simulink model "s3_c2_luenberger"  (R2023a)
settings: Solver=FixedStepAuto  StartTime=0.0  StopTime=32  FixedStep=1E-3  RelTol=1e-3
undefined symbols (not defined in the file): A, A_c2, B1, C, C_obs1, C_obs2, CI, Ko1_luenberger, Ko2_luenberger
settings Model: Creator=felipe  LastModifiedBy=felipe

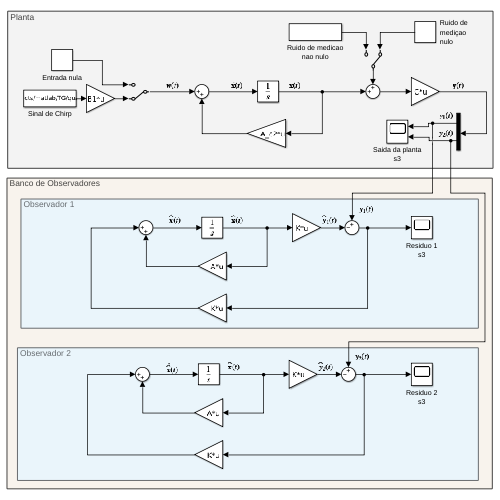
[thumbnail: Simulink's stored preview of the top-level diagram]
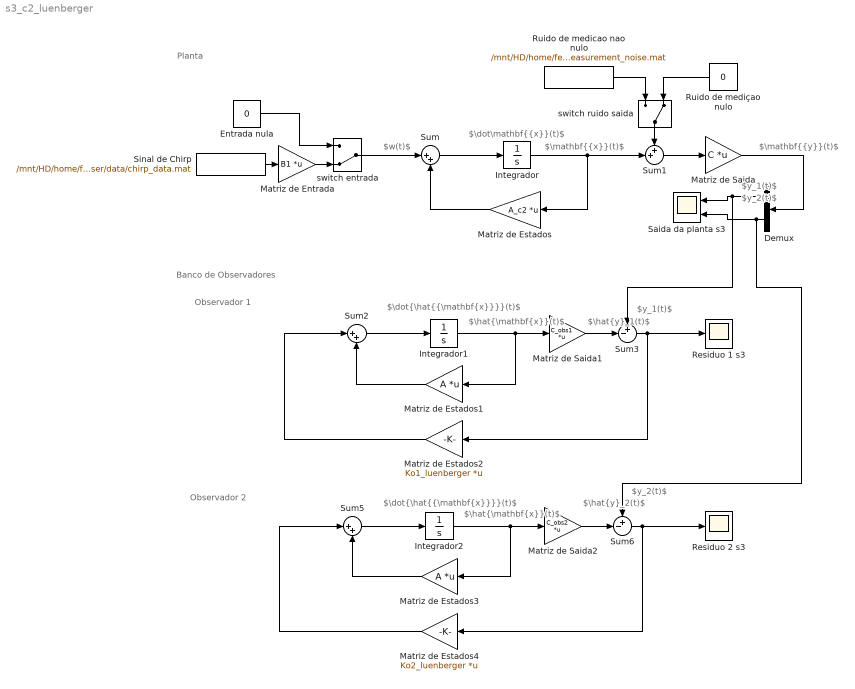
== system s3_c2_luenberger ==
  note: $\dot{\hat{{\mathbf{x}}}}(t)$
  note: Banco de Observadores
  note: Observador 1
  note: $w(t)$
  note: Planta
  note: $\dot\mathbf{{x}}(t)$
  note: $\mathbf{{x}}(t)$
  note: $\mathbf{{y}}(t)$
  note: Observador 2
  note: $y_1(t)$
  note: $y_2(t)$
  note: $\hat{y}_1(t)$
  note: $\hat{\mathbf{x}}(t)$
  note: $\dot{\hat{{\mathbf{x}}}}(t)$
  note: $\hat{y}_2(t)$
  note: $\hat{\mathbf{x}}(t)$
  note: $y_1(t)$
  note: $y_2(t)$
  Demux : Demux  Outputs=2
  Entrada nula : Constant  Value=0
  Integrador : Integrator  InitialCondition=CI
  Integrador1 : Integrator
  Integrador2 : Integrator
  Matriz de Entrada : Gain  Gain=B1  Multiplication=Matrix(K*u)
  Matriz de Estados : Gain  Gain=A_c2  Multiplication=Matrix(K*u)
  Matriz de Estados1 : Gain  Gain=A  Multiplication=Matrix(K*u)
  Matriz de Estados2 : Gain  Gain=Ko1_luenberger  Multiplication=Matrix(K*u)
  Matriz de Estados3 : Gain  Gain=A  Multiplication=Matrix(K*u)
  Matriz de Estados4 : Gain  Gain=Ko2_luenberger  Multiplication=Matrix(K*u)
  Matriz de Saida : Gain  Gain=C  Multiplication=Matrix(K*u)
  Matriz de Saida1 : Gain  Gain=C_obs1  Multiplication=Matrix(K*u)
  Matriz de Saida2 : Gain  Gain=C_obs2  Multiplication=Matrix(K*u)
  Residuo 1 s3 : Scope
  Residuo 2 s3 : Scope
  Ruido de mediçao nulo : Constant  Value=0
  Ruido de medicao nao nulo : FromFile  FileName=/mnt/HD/home/felipe/Projects/matlab/TG/quanser/data/measurement_noise.mat  SampleTime=0
  Saida da planta s3 : Scope  NumInputPorts=2
  Sinal de Chirp : FromFile  FileName=/mnt/HD/home/felipe/Projects/matlab/TG/quanser/data/chirp_data.mat  SampleTime=0
  Sum : Sum  Inputs=|++
  Sum1 : Sum  Inputs=++|
  Sum2 : Sum  Inputs=|++
  Sum3 : Sum  Inputs=+-|
  Sum5 : Sum  Inputs=|++
  Sum6 : Sum  Inputs=+-|
  switch entrada : ManualSwitch  CurrentSetting=0
  switch ruido saida : ManualSwitch  CurrentSetting=0
  wires:
  Sum/1 -> Integrador/1
  Matriz de Estados/1 -> Sum/2
  Integrador/1 -> Sum1/2, Matriz de Estados/1
  Matriz de Saida/1 -> Demux/1
  Sinal de Chirp/1 -> Matriz de Entrada/1
  Matriz de Entrada/1 -> switch entrada/2
  Entrada nula/1 -> switch entrada/1
  Sum1/1 -> Matriz de Saida/1
  switch ruido saida/1 -> Sum1/1
  Ruido de mediçao nulo/1 -> switch ruido saida/2
  Ruido de medicao nao nulo/1 -> switch ruido saida/1
  switch entrada/1 -> Sum/1
  Sum3/1 -> Matriz de Estados2/1, Residuo 1 s3/1
  Integrador1/1 -> Matriz de Saida1/1, Matriz de Estados1/1
  Sum2/1 -> Integrador1/1
  Matriz de Estados1/1 -> Sum2/2
  Matriz de Saida1/1 -> Sum3/2
  Matriz de Estados2/1 -> Sum2/1
  Demux/1 -> Sum3/1, Saida da planta s3/1
  Integrador2/1 -> Matriz de Saida2/1, Matriz de Estados3/1
  Matriz de Estados4/1 -> Sum5/1
  Matriz de Estados3/1 -> Sum5/2
  Sum6/1 -> Residuo 2 s3/1, Matriz de Estados4/1
  Sum5/1 -> Integrador2/1
  Matriz de Saida2/1 -> Sum6/2
  Demux/2 -> Saida da planta s3/2, Sum6/1
